simulink model "lab02fig02"  (R2015a)
settings: Solver=ode45  StartTime=0.0  StopTime=50.0  RelTol=1e-3
settings Model: Creator=dg  LastModifiedBy=dg

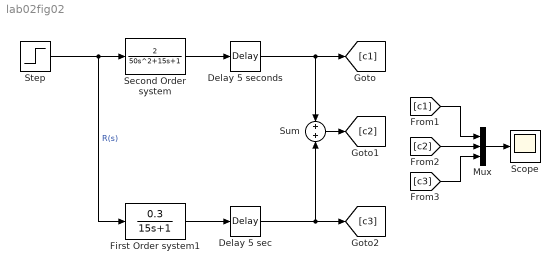
== system lab02fig02 ==
  Delay 5 seconds : TransportDelay  DelayTime=5
  Delay 5 sec : TransportDelay  DelayTime=5
  First Order system1 : TransferFcn  Numerator=[0.3]  Denominator=[15 1]
  Mux : Mux  Inputs=3
  Scope : Scope
      settings: YMin=-1  YMax=1
  Second Order system : TransferFcn  Numerator=[2]  Denominator=[50 15 1]
  Step : Step  Time=0  SampleTime=0
  Sum : Sum  Inputs=+|+
  wires:
  Step/1 -> First Order system1/1, Second Order system/1  "R(s)"
  Second Order system/1 -> Delay 5 seconds/1
  [c1] -> Mux/1
  [c2] -> Mux/2
  [c3] -> Mux/3
  Mux/1 -> Scope/1
  Delay 5 seconds/1 -> [c1], Sum/1
  Sum/1 -> [c2]
  First Order system1/1 -> Delay 5 sec/1
  Delay 5 sec/1 -> Sum/2, [c3]
